simulink model "ContinousControl"  (R2021b)
settings: Solver=ode4  StartTime=0.0  StopTime=SIM_TIME  FixedStep=SIM_STEP  RelTol=1e-3
undefined symbols (not defined in the file): A, B, C, K, x0
settings Model: Creator=tanzc  LastModifiedBy=tanzc
settings DataIOCC: SaveFormat=Array  ReturnWorkspaceOutputs=off

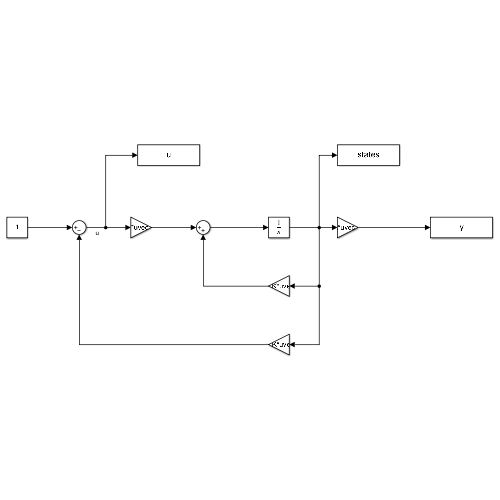
[thumbnail: Simulink's stored preview of the top-level diagram]
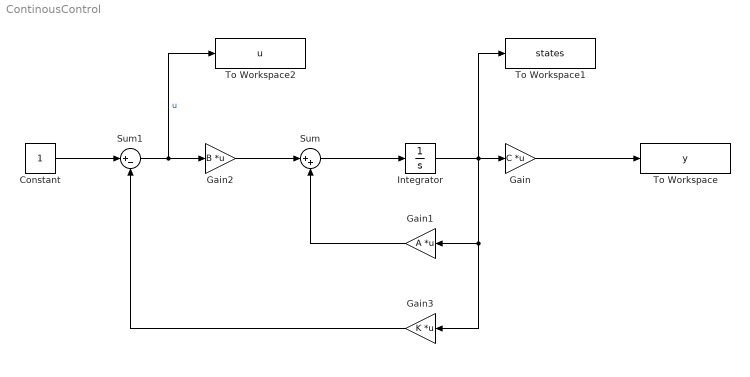
== system ContinousControl ==
  Constant : Constant
  Gain : Gain  Gain=C  Multiplication=Matrix(K*u) (u vector)
  Gain1 : Gain  Gain=A  Multiplication=Matrix(K*u) (u vector)
  Gain2 : Gain  Gain=B  Multiplication=Matrix(K*u) (u vector)
  Gain3 : Gain  Gain=K  Multiplication=Matrix(K*u) (u vector)
  Integrator : Integrator  InitialCondition=x0
  Sum : Sum  Inputs=|++
  Sum1 : Sum  Inputs=|+-
  To Workspace : ToWorkspace  VariableName=y  SaveFormat=Timeseries  SampleTime=-1
  To Workspace1 : ToWorkspace  VariableName=states  SaveFormat=Timeseries  SampleTime=-1
  To Workspace2 : ToWorkspace  VariableName=u  SaveFormat=Timeseries  SampleTime=-1
  wires:
  Sum1/1 -> To Workspace2/1, Gain2/1  "u"
  Gain2/1 -> Sum/1
  Gain1/1 -> Sum/2
  Gain/1 -> To Workspace/1
  Sum/1 -> Integrator/1
  Constant/1 -> Sum1/1
  Integrator/1 -> To Workspace1/1, Gain3/1, Gain1/1, Gain/1
  Gain3/1 -> Sum1/2
